simulink model "Lab3model"  (R2024b)
settings: Solver=VariableStepAuto  StartTime=0.0  StopTime=10.0  RelTol=1e-3
undefined symbols (not defined in the file): K, tau, To
libraries: simulink_extras x2
settings Model: Creator=emersonhall  LastModifiedBy=emersonhall

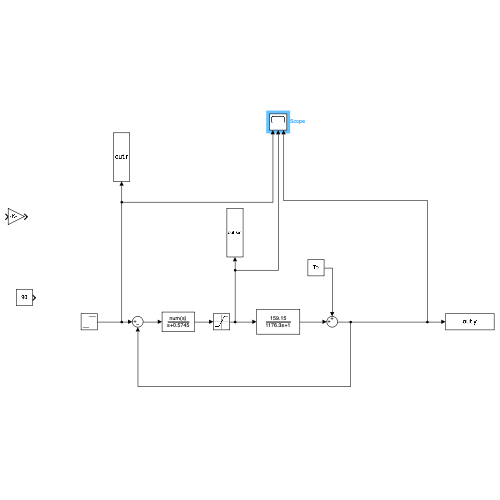
[thumbnail: Simulink's stored preview of the top-level diagram]
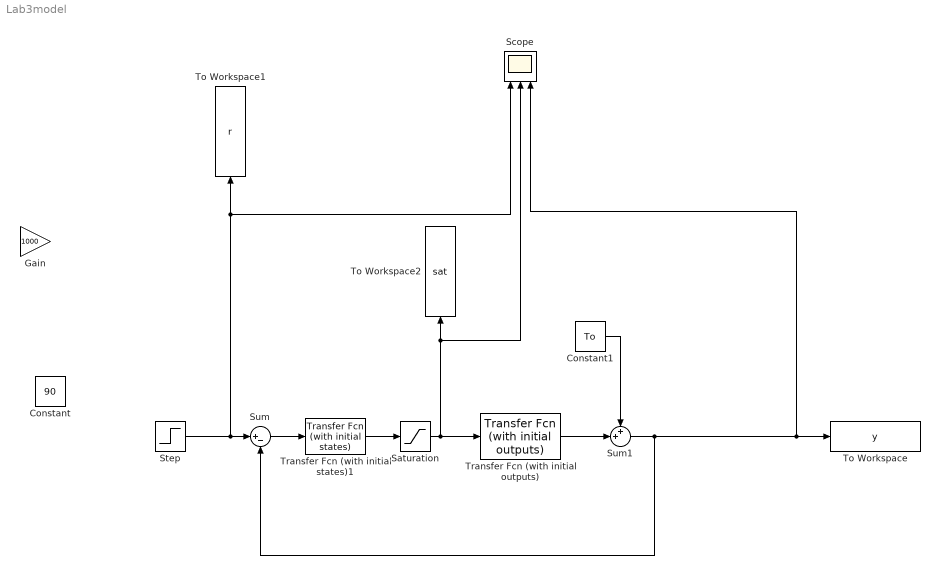
== system Lab3model ==
  Constant : Constant  Value=90
  Constant1 : Constant  Value=To
  Gain : Gain  Gain=1000
  Saturation : Saturate  UpperLimit=100  LowerLimit=0
  Scope : Scope  NumInputPorts=3
  Step : Step  Time=0.5  After=90  SampleTime=0
  Sum : Sum  Inputs=|+-
  Sum1 : Sum  Inputs=++|
  To Workspace : ToWorkspace  VariableName=y  SaveFormat=Timeseries  SampleTime=-1
  To Workspace1 : ToWorkspace  VariableName=r  SaveFormat=Timeseries  SampleTime=-1
  To Workspace2 : ToWorkspace  VariableName=sat  SaveFormat=Timeseries  SampleTime=-1
  Transfer Fcn (with initial outputs) : simulink_extras/Additional Linear/Transfer Fcn (with initial outputs)  N=[K]  D="[tau  1]"  Y0=0  U0=0
  Transfer Fcn (with initial states)1 : simulink_extras/Additional Linear/Transfer Fcn (with initial states)  N=[21.604 13.804956]  D="[1  0.5745]"  X0=.5
  wires:
  Saturation/1 -> Scope/2, To Workspace2/1, Transfer Fcn (with initial outputs)/1
  Transfer Fcn (with initial outputs)/1 -> Sum1/2
  Constant1/1 -> Sum1/1
  Sum1/1 -> Scope/3, To Workspace/1, Sum/2
  Step/1 -> Sum/1, Scope/1, To Workspace1/1
  Transfer Fcn (with initial states)1/1 -> Saturation/1
  Sum/1 -> Transfer Fcn (with initial states)1/1
